simulink library "flapping_dynamics"  (R2022b)
settings: Solver=VariableStepAuto  StartTime=0.0  StopTime=10.0  RelTol=1e-3
undefined symbols (not defined in the file or in its folder): plant_sample_time_s, veh_params
settings Model: Creator=Tanmay.Mandal  LastModifiedBy=Tanmay.Mandal

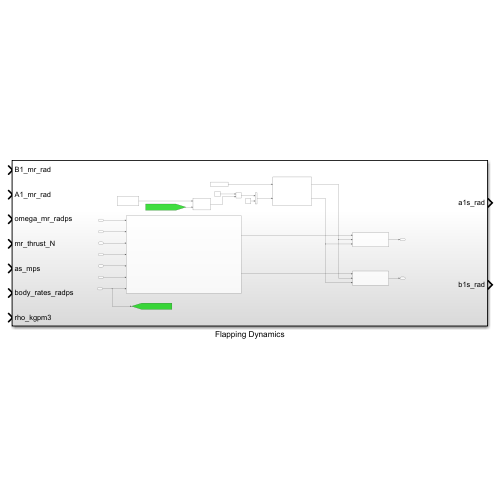
[thumbnail: Simulink's stored preview of the top-level diagram]
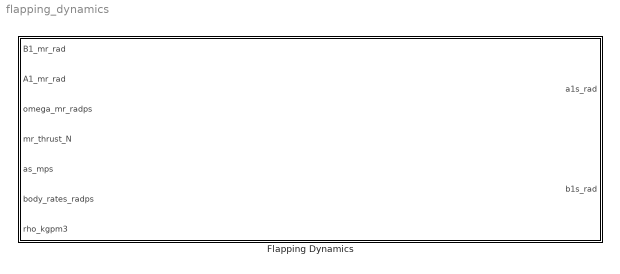
== system flapping_dynamics ==
  Flapping Dynamics : Subsystem

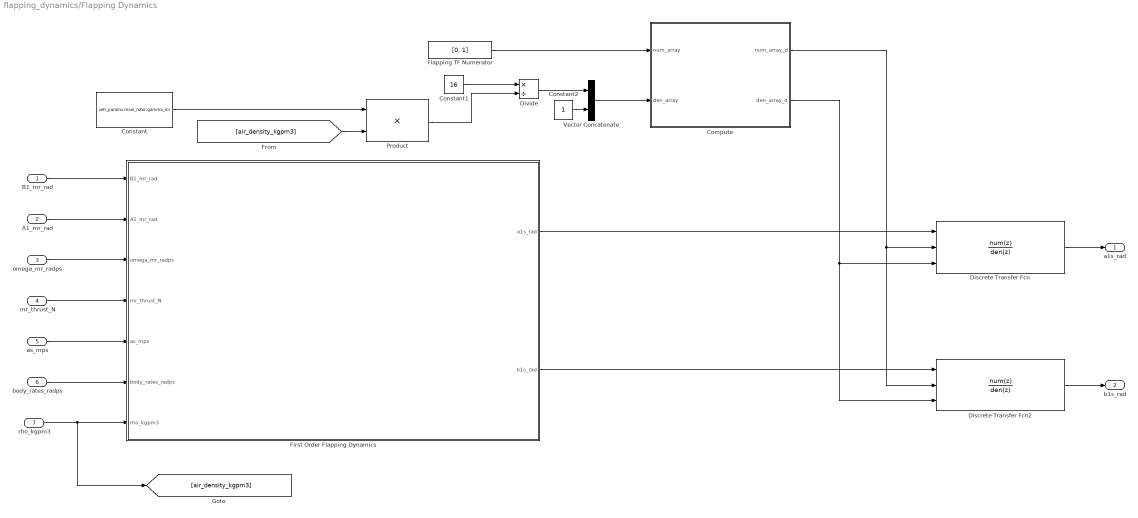
== system flapping_dynamics/Flapping Dynamics ==
  B1_mr_rad : Inport
  A1_mr_rad : Inport  Port=2
  omega_mr_radps : Inport  Port=3
  mr_thrust_N : Inport  Port=4
  as_mps : Inport  Port=5
  body_rates_radps : Inport  Port=6
  rho_kgpm3 : Inport  Port=7
  Compute : MATLAB Function  TreatAsAtomicUnit=on  mask{sample_time_s=plant_sample_time_s}
      mask prompts: sample_time_s "Sample Time [sec]"
  Constant : Constant  Value=veh_params.main_rotor.gamma_mr  SampleTime=plant_sample_time_s
  Constant1 : Constant  Value=16  SampleTime=plant_sample_time_s
  Constant2 : Constant
  Discrete Transfer Fcn : DiscreteTransferFcn  NumeratorSource=Input port  DenominatorSource=Input port  SampleTime=plant_sample_time_s  a0EqualsOne=on
      settings: InputPortMap=u0,p1,p3
  Discrete Transfer Fcn2 : DiscreteTransferFcn  NumeratorSource=Input port  DenominatorSource=Input port  SampleTime=plant_sample_time_s  a0EqualsOne=on
      settings: InputPortMap=u0,p1,p3
  Divide : Product  Inputs=*/
  First Order Flapping Dynamics : MATLAB Function  TreatAsAtomicUnit=on  mask{params=veh_params.main_rotor}
      mask prompts: params "Main Rotor Params Struct"
  Flapping TF Numerator : Constant  Value=[0, 1]  SampleTime=plant_sample_time_s
  Product : Product
  Vector Concatenate : Concatenate
  a1s_rad : Outport
  b1s_rad : Outport  Port=2
  wires:
  B1_mr_rad/1 -> First Order Flapping Dynamics/1(B1_mr_rad)
  First Order Flapping Dynamics/1(a1s_rad) -> Discrete Transfer Fcn/1
  omega_mr_radps/1 -> First Order Flapping Dynamics/3(omega_mr_radps)
  A1_mr_rad/1 -> First Order Flapping Dynamics/2(A1_mr_rad)
  rho_kgpm3/1 -> [air_density_kgpm3], First Order Flapping Dynamics/7(rho_kgpm3)
  as_mps/1 -> First Order Flapping Dynamics/5(as_mps)
  body_rates_radps/1 -> First Order Flapping Dynamics/6(body_rates_radps)
  mr_thrust_N/1 -> First Order Flapping Dynamics/4(mr_thrust_N)
  First Order Flapping Dynamics/2(b1s_rad) -> Discrete Transfer Fcn2/1
  Discrete Transfer Fcn/1 -> a1s_rad/1
  Discrete Transfer Fcn2/1 -> b1s_rad/1
  Compute/1(num_array_d) -> Discrete Transfer Fcn2/2, Discrete Transfer Fcn/2
  Compute/2(den_array_d) -> Discrete Transfer Fcn2/3, Discrete Transfer Fcn/3
  Flapping TF Numerator/1 -> Compute/1(num_array)
  Constant/1 -> Product/1
  Product/1 -> Divide/2
  Vector Concatenate/1 -> Compute/2(den_array)
  [air_density_kgpm3] -> Product/2
  Constant1/1 -> Divide/1
  Divide/1 -> Vector Concatenate/1
  Constant2/1 -> Vector Concatenate/2

== matlab function flapping_dynamics/Flapping Dynamics/Compute ==
  data: num_array input; num_array_d output; den_array input; den_array_d output; sample_time_s parameter
function [num_array_d, den_array_d] = compute_discrete_tf(num_array, den_array, sample_time_s)
%COMPUTE_DISCRETE_TF For a given numerator and denominator of the
% first order continuous transfer function this function computes the numerator and
% denominator of the corresponding discrete transfer function using Tustin
% transformation
%
%Inputs:
%num_array              : Numerator of the TF in the form (B1*s + B0)/(A1*s + A0)
%den_array              : Denominator of the TF
%sample_time_s          : Sample time in seconds
%
%Outputs:
%num_array_d            : Numerator of the discrete TF in the form b0 + b1*z^-1/a0 + a1*z^-1
%den_array_d            : Denominator of the discrete TF
[num_array_d, den_array_d] = cont_to_discrete_1st_order_tf(num_array, den_array, sample_time_s);
end

== matlab function flapping_dynamics/Flapping Dynamics/First Order Flapping Dynamics ==
  data: B1_mr_rad input; a1s_rad output size=1; A1_mr_rad input; omega_mr_radps input; mr_thrust_N input; as_mps input; body_rates_radps input; rho_kgpm3 input; b1s_rad output size=1; params parameter
function [a1s_rad, b1s_rad] = first_order_flapping_mr(B1_mr_rad, A1_mr_rad, omega_mr_radps, ...
                       mr_thrust_N, as_mps, body_rates_radps, rho_kgpm3, params)
%FIRST_ORDER_FLAPPING_MR implements first order flapping dynamics
%for the main rotor. A steady state assumption is used, which assumes
%that tip path plane (TPP) changes it's orientation instantaneously
%(transient flap motion is highly damped with time constant of approx
%16/gamma_mr). This implies transient response dies out after less than one
%revolution of the main rotor. Therefore a1dot = b1dot = 0. Where a1dot and
%b1dot is measured w.r.t to swash plate
%
%Inputs:
%B1_mr_rad          :       Cyclic pitch input
%A1_mr_rad          :       Cyclic roll input
%omega_mr_radps     :       Angular velocity of the main rotor
%mr_thrust_N        :       Rotor thrust from previous iteration
%as_mps             :       Airspeed (3D)
%body_rates_mps     :       Body angular rates
%rho_kgpm3          :       Air Density
%params             :       Main rotor and vehicle parameters struct
%
%Outputs:
%a1s_rad            :       Main rotor longitudinal tilt w.r.t to hub plane
%b1s_rad            :       Main rotor lateral tilt w.r.t to hub plane
[a1s_rad, b1s_rad] = first_order_flapping_mr_function(B1_mr_rad, A1_mr_rad, omega_mr_radps, ...
                       mr_thrust_N, as_mps, body_rates_radps, rho_kgpm3, params);
end
